simulink model "motor_model_final"  (R2020a)
settings: Solver=VariableStepAuto  StartTime=0.0  StopTime=20  RelTol=1e-3
undefined symbols (not defined in the file or in its folder): ctrl_deadZone, k_motor, Km, L, Motor, Motor_Lib, R, sigbuilder_block, X, Y, Z
libraries: fl_lib x45, nesl_utility x36, ee_lib x9, sm_lib x8, sdl_lib x3, simulink x1
(part 2 of 2)

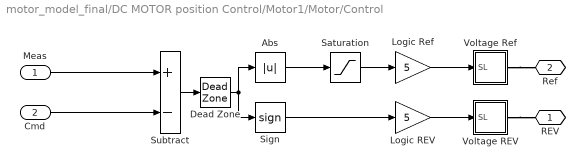
== system motor_model_final/DC MOTOR position Control/Motor1/Motor/Control ==
  Meas : Inport  RequirementInfo={} %GIDa_619c2803_28d3_4ef7_ba70_833e220e126d
  Cmd : Inport  RequirementInfo={} %GIDa_cedc12fc_cc18_42d0_9a71_21d4f8b9a5ca  Port=2
  Abs : Abs  RequirementInfo={} %GIDa_d0313f18_77fc_4469_88ee_421a3cb03dd3  ZeroCross=off
  Dead Zone : DeadZone  RequirementInfo={} %GIDa_8c142244_20db_463a_b94f_674c218bd698  LowerValue=-ctrl_deadZone  UpperValue=ctrl_deadZone  ZeroCross=off  SaturateOnIntegerOverflow=on
  Logic REV : Gain  RequirementInfo={} %GIDa_b932483c_9411_4fcb_821f_6d68825134f0  Gain=5
  Logic Ref : Gain  RequirementInfo={} %GIDa_11f4073f_f2f5_4fa6_a867_14315e93e3df  Gain=5
  Saturation : Saturate  UpperLimit=1  LowerLimit=0  ZeroCross=off
  Sign : Signum  RequirementInfo={} %GIDa_d20f7fe8_60b8_4a21_b668_3ad824d4ede9  ZeroCross=off
  Subtract : Sum  RequirementInfo={} %GIDa_19bf5a43_019a_4db9_b97f_957f1fcc13e1  Inputs=+-
  Voltage REV : Subsystem  RequirementInfo={} %GIDa_c0e87e75_602b_4cdc_bd7f_8168c58f4b38
  Voltage Ref : Subsystem  RequirementInfo={} %GIDa_8f8c4948_8993_460a_8a8e_45d690a1b1f5
  REV : PMIOPort  RequirementInfo={} %GIDa_bf5c9ce0_d82a_4963_bef4_f9b0d83d66de  Side=Right
  Ref : PMIOPort  RequirementInfo={} %GIDa_1cf45b29_5f52_4f47_a585_a1bd10a239a7  Port=2  Side=Right
  wires:
  Saturation/1 -> Logic Ref/1
  Meas/1 -> Subtract/1
  Abs/1 -> Saturation/1
  Sign/1 -> Logic REV/1
  Logic REV/1 -> Voltage REV/1(SL)
  Cmd/1 -> Subtract/2
  Logic Ref/1 -> Voltage Ref/1(SL)
  Subtract/1 -> Dead Zone/1
  Dead Zone/1 -> Abs/1, Sign/1
  connections:
  Voltage Ref/RConn1 -- Ref/RConn1
  Voltage REV/RConn1 -- REV/RConn1

== system motor_model_final/DC MOTOR position Control/Motor1/Motor/Network ==
  Abs : Abs  ZeroCross=off
  Current Sensor : fl_lib/Electrical/Electrical Sensors/Current Sensor  RequirementInfo={} %GIDa_513c3105_2bac_45e4_b484_9e853d23afd7
  Current Source : fl_lib/Electrical/Electrical Sources/Controlled Current Source  RequirementInfo={} %GIDa_94a24adf_c038_4ce1_83ad_37f20f638e14
  ERef : fl_lib/Electrical/Electrical Elements/Electrical Reference
  PS-Simulink Converter : nesl_utility/PS-Simulink Converter  PhysicalDomain=network_engine_domain  SubClassName=ps_output  LeftPortType=input  RightPortType=output  PseudoPeriodic=off  Frequencies=[]  Unit=1  AffineConversion=off
  Simulink-PS Converter : nesl_utility/Simulink-PS Converter  PhysicalDomain=network_engine_domain  SubClassName=ps_input  LeftPortType=input  RightPortType=output  PseudoPeriodic=off  Frequencies=[]  NoiseDistribution=none  NoiseParameters=[]  Unit=1  AffineConversion=off  FilteringAndDerivatives=zero  SimscapeFilterOrder=1  InputFilterTimeConstant=0.005  UdotUserProvided=1
  " M" : PMIOPort  RequirementInfo={} %GIDa_84871c60_653c_4020_b9b8_d9b6ede8c9f6  Side=Left
  - : PMIOPort  RequirementInfo={} %GIDa_c912cfdd_b223_4c72_a577_976fa4621da7  Port=2  Side=Right
  + : PMIOPort  RequirementInfo={} %GIDa_bf626ff5_1ed8_4472_be8d_8f3179a83c03  Port=3  Side=Left
  wires:
  Abs/1 -> Simulink-PS Converter/1
  PS-Simulink Converter/1 -> Abs/1
  connections:
  Simulink-PS Converter/RConn1 -- Current Source/RConn1
  ERef/LConn1 -- Current Sensor/RConn2
  " M"/RConn1 -- Current Sensor/LConn1
  Current Sensor/RConn1 -- PS-Simulink Converter/LConn1
  +/RConn1 -- Current Source/RConn2
  -/RConn1 -- Current Source/LConn1

== system motor_model_final/DC MOTOR position Control/Motor1/Motor/Rotational Simscape Intf ==
  Angular Velocity Source : fl_lib/Mechanical/Mechanical Sources/Ideal Angular Velocity Source  RequirementInfo={} %GIDa_9c63d25c_cbc1_48c9_8ca4_1c1f53bf651e
  Torque Sensor : fl_lib/Mechanical/Mechanical Sensors/Ideal Torque Sensor  RequirementInfo={} %GIDa_cf1090dc_72bf_4751_af0a_ba0ab775e595
  w : PMIOPort  RequirementInfo={} %GIDa_f25d5e0a_0e94_4d54_ac21_7ad0e7ab5701  Side=Right
  t : PMIOPort  RequirementInfo={} %GIDa_028763a7_4726_4672_beaf_1abf56a90cfd  Port=2  Side=Left
  R : PMIOPort  RequirementInfo={} %GIDa_22d96cb3_e01c_43f5_a1b0_795c055d4914  Port=3  Side=Left
  C : PMIOPort  RequirementInfo={} %GIDa_120a4565_964d_4dd8_b46f_0df667ed0ae0  Port=4  Side=Right
  connections:
  Torque Sensor/RConn1 -- C/RConn1
  R/RConn1 -- Angular Velocity Source/LConn1
  Torque Sensor/LConn1 -- Angular Velocity Source/RConn2
  t/RConn1 -- Torque Sensor/RConn2
  w/RConn1 -- Angular Velocity Source/RConn1

== system motor_model_final/DC MOTOR PWM Control/Motor1/Motor/Control/Voltage REV ==
  SL : Inport
  Controlled Voltage Source : fl_lib/Electrical/Electrical Sources/Controlled Voltage Source
  ERef : fl_lib/Electrical/Electrical Elements/Electrical Reference
  Simulink-PS Converter : nesl_utility/Simulink-PS Converter  PhysicalDomain=network_engine_domain  SubClassName=ps_input  LeftPortType=input  RightPortType=output  PseudoPeriodic=off  Frequencies=[]  NoiseDistribution=none  NoiseParameters=[]  Unit=V  AffineConversion=off  FilteringAndDerivatives=zero  SimscapeFilterOrder=1  InputFilterTimeConstant=0.005  UdotUserProvided=0
  V : PMIOPort  Side=Right
  wires:
  SL/1 -> Simulink-PS Converter/1
  connections:
  ERef/LConn1 -- Controlled Voltage Source/RConn2
  V/RConn1 -- Controlled Voltage Source/LConn1
  Simulink-PS Converter/RConn1 -- Controlled Voltage Source/RConn1

== system motor_model_final/DC MOTOR PWM Control/Motor1/Motor/Control/Voltage Ref ==
  SL : Inport
  Controlled Voltage Source : fl_lib/Electrical/Electrical Sources/Controlled Voltage Source
  ERef : fl_lib/Electrical/Electrical Elements/Electrical Reference
  Simulink-PS Converter : nesl_utility/Simulink-PS Converter  PhysicalDomain=network_engine_domain  SubClassName=ps_input  LeftPortType=input  RightPortType=output  PseudoPeriodic=off  Frequencies=[]  NoiseDistribution=none  NoiseParameters=[]  Unit=V  AffineConversion=off  FilteringAndDerivatives=zero  SimscapeFilterOrder=1  InputFilterTimeConstant=0.005  UdotUserProvided=0
  V : PMIOPort  Side=Right
  wires:
  SL/1 -> Simulink-PS Converter/1
  connections:
  Simulink-PS Converter/RConn1 -- Controlled Voltage Source/RConn1
  V/RConn1 -- Controlled Voltage Source/LConn1
  ERef/LConn1 -- Controlled Voltage Source/RConn2

== system motor_model_final/DC MOTOR Speed Control/Motor1/Motor/Control/Voltage REV ==
  SL : Inport
  Controlled Voltage Source : fl_lib/Electrical/Electrical Sources/Controlled Voltage Source
  ERef : fl_lib/Electrical/Electrical Elements/Electrical Reference
  Simulink-PS Converter : nesl_utility/Simulink-PS Converter  PhysicalDomain=network_engine_domain  SubClassName=ps_input  LeftPortType=input  RightPortType=output  PseudoPeriodic=off  Frequencies=[]  NoiseDistribution=none  NoiseParameters=[]  Unit=V  AffineConversion=off  FilteringAndDerivatives=zero  SimscapeFilterOrder=1  InputFilterTimeConstant=0.005  UdotUserProvided=0
  V : PMIOPort  Side=Right
  wires:
  SL/1 -> Simulink-PS Converter/1
  connections:
  ERef/LConn1 -- Controlled Voltage Source/RConn2
  V/RConn1 -- Controlled Voltage Source/LConn1
  Simulink-PS Converter/RConn1 -- Controlled Voltage Source/RConn1

== system motor_model_final/DC MOTOR Speed Control/Motor1/Motor/Control/Voltage Ref ==
  SL : Inport
  Controlled Voltage Source : fl_lib/Electrical/Electrical Sources/Controlled Voltage Source
  ERef : fl_lib/Electrical/Electrical Elements/Electrical Reference
  Simulink-PS Converter : nesl_utility/Simulink-PS Converter  PhysicalDomain=network_engine_domain  SubClassName=ps_input  LeftPortType=input  RightPortType=output  PseudoPeriodic=off  Frequencies=[]  NoiseDistribution=none  NoiseParameters=[]  Unit=V  AffineConversion=off  FilteringAndDerivatives=zero  SimscapeFilterOrder=1  InputFilterTimeConstant=0.005  UdotUserProvided=0
  V : PMIOPort  Side=Right
  wires:
  SL/1 -> Simulink-PS Converter/1
  connections:
  Simulink-PS Converter/RConn1 -- Controlled Voltage Source/RConn1
  V/RConn1 -- Controlled Voltage Source/LConn1
  ERef/LConn1 -- Controlled Voltage Source/RConn2

== system motor_model_final/DC MOTOR position Control/Motor1/Motor/Control/Voltage REV ==
  SL : Inport  RequirementInfo={} %GIDa_dea8ea81_1710_4fb8_ba02_6f2c02265479
  Controlled Voltage Source : fl_lib/Electrical/Electrical Sources/Controlled Voltage Source  RequirementInfo={} %GIDa_18b8d214_2427_4381_a540_d572da4e9001
  ERef : fl_lib/Electrical/Electrical Elements/Electrical Reference  RequirementInfo={} %GIDa_462338b2_4d7f_47c7_89f7_87b59660760b
  Simulink-PS Converter : nesl_utility/Simulink-PS Converter  RequirementInfo={} %GIDa_0fb8daf5_cf0e_41aa_bdfd_c463d772de6d  PhysicalDomain=network_engine_domain  SubClassName=ps_input  LeftPortType=input  RightPortType=output  PseudoPeriodic=off  Frequencies=[]  NoiseDistribution=none  NoiseParameters=[]  Unit=V  AffineConversion=off  FilteringAndDerivatives=zero  SimscapeFilterOrder=1  InputFilterTimeConstant=0.005  UdotUserProvided=0
  V : PMIOPort  RequirementInfo={} %GIDa_c42b8280_047e_43ce_ada1_0ab47814a1ff  Side=Right
  wires:
  SL/1 -> Simulink-PS Converter/1
  connections:
  Simulink-PS Converter/RConn1 -- Controlled Voltage Source/RConn1
  V/RConn1 -- Controlled Voltage Source/LConn1
  ERef/LConn1 -- Controlled Voltage Source/RConn2

== system motor_model_final/DC MOTOR position Control/Motor1/Motor/Control/Voltage Ref ==
  SL : Inport  RequirementInfo={} %GIDa_419a7471_849d_441c_84b1_4e25bcdc027c
  Controlled Voltage Source : fl_lib/Electrical/Electrical Sources/Controlled Voltage Source  RequirementInfo={} %GIDa_6e64d9cc_3e6c_4d3a_a6fc_3228a91425c7
  ERef : fl_lib/Electrical/Electrical Elements/Electrical Reference  RequirementInfo={} %GIDa_884cea57_6d0e_4e6b_b934_7eb0c59af366
  Simulink-PS Converter : nesl_utility/Simulink-PS Converter  RequirementInfo={} %GIDa_7c09949d_fb09_4c67_b267_9eeb2ab661fd  PhysicalDomain=network_engine_domain  SubClassName=ps_input  LeftPortType=input  RightPortType=output  PseudoPeriodic=off  Frequencies=[]  NoiseDistribution=none  NoiseParameters=[]  Unit=V  AffineConversion=off  FilteringAndDerivatives=zero  SimscapeFilterOrder=1  InputFilterTimeConstant=0.005  UdotUserProvided=0
  V : PMIOPort  RequirementInfo={} %GIDa_06de9ff4_dfb2_4b63_b424_d78d422e5b2d  Side=Right
  wires:
  SL/1 -> Simulink-PS Converter/1
  connections:
  ERef/LConn1 -- Controlled Voltage Source/RConn2
  V/RConn1 -- Controlled Voltage Source/LConn1
  Simulink-PS Converter/RConn1 -- Controlled Voltage Source/RConn1
